simulink model "altitude_loop"  (Simulink 8.2)
settings: Solver=ode45  StartTime=0.0  StopTime=500  RelTol=1e-3
undefined symbols (not defined in the file): P
settings Model: Creator=paul  LastModifiedBy=paul
settings DataIOCC: SignalLoggingSaveFormat=Dataset
settings OptimizationCC: ExpressionDepthLimit=128
settings DebuggingCC: FcnCallInpInsideContextMsg=EnableAllAsError  StateNameClashWarn=none
settings GRTTargetCC: CombineOutputUpdateFcns=on  GRTInterface=off

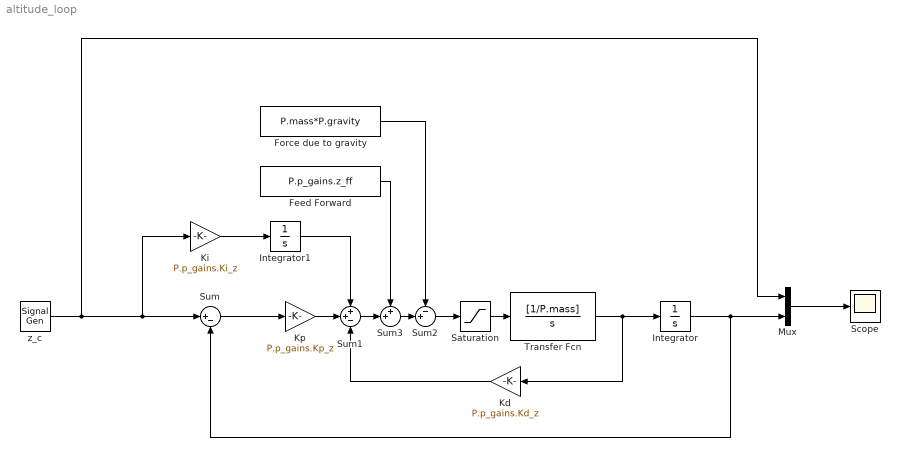
== system altitude_loop ==
  Feed Forward : Constant  Value=P.p_gains.z_ff
  Force due to gravity : Constant  Value=P.mass*P.gravity
  Integrator : Integrator
  Integrator1 : Integrator
  Kd : Gain  Gain=P.p_gains.Kd_z
  Ki : Gain  Gain=P.p_gains.Ki_z
  Kp : Gain  Gain=P.p_gains.Kp_z
  Mux : Mux  Inputs=2
  Saturation : Saturate  UpperLimit=P.F_max  LowerLimit=0
  Scope : Scope
  Sum : Sum  Inputs=|+-
  Sum1 : Sum  Inputs=++-
  Sum2 : Sum  Inputs=-+|
  Sum3 : Sum  Inputs=++|
  Transfer Fcn : TransferFcn  Numerator=[1/P.mass]  Denominator=[1 0]
  z_c : SignalGenerator  WaveForm=square  Amplitude=0.5  Frequency=0.05  Units=rad/sec
  wires:
  Mux/1 -> Scope/1
  z_c/1 -> Ki/1, Sum/1, Mux/1
  Force due to gravity/1 -> Sum2/1
  Feed Forward/1 -> Sum3/1
  Sum2/1 -> Saturation/1
  Saturation/1 -> Transfer Fcn/1
  Sum3/1 -> Sum2/2
  Transfer Fcn/1 -> Kd/1, Integrator/1
  Integrator1/1 -> Sum1/1
  Kd/1 -> Sum1/3
  Kp/1 -> Sum1/2
  Sum1/1 -> Sum3/2
  Ki/1 -> Integrator1/1
  Sum/1 -> Kp/1
  Integrator/1 -> Mux/2, Sum/2
